simulink model "Task2"  (R2018a)
settings: Solver=FixedStepAuto  StartTime=0.0  StopTime=20  FixedStep=0.01  RelTol=1e-3
libraries: fl_lib x11, nesl_utility x7, simulink x3, elec_lib x3, sdl_lib x1
settings Model: Creator=Archana  LastModifiedBy=samak

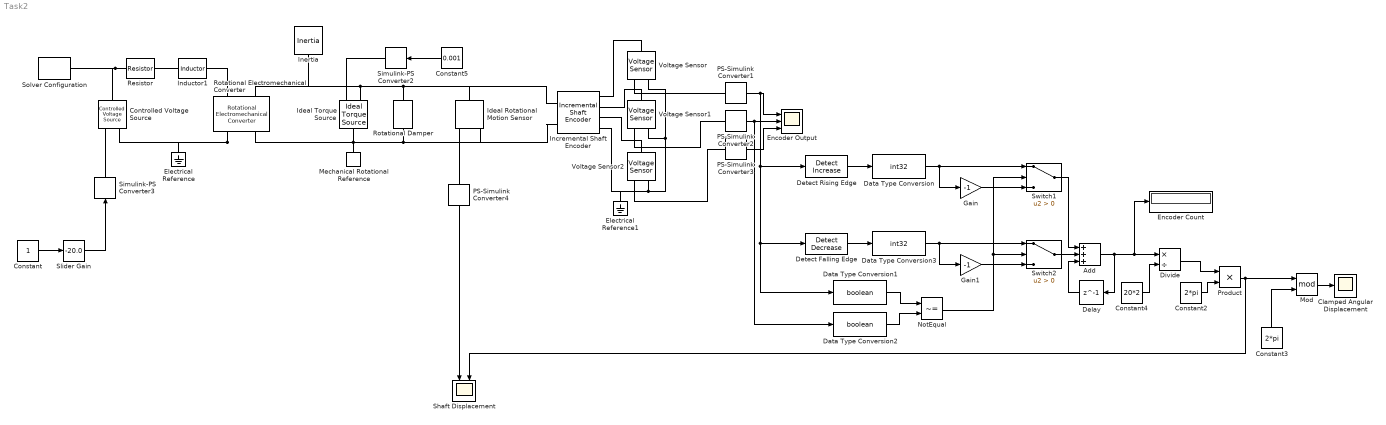
== system Task2 ==
  Add : Sum  Inputs=+++
  Clamped Angular Displacement : Scope
  "Constant " : Constant
  Constant2 : Constant  Value=2*pi
  Constant3 : Constant  Value=2*pi
  Constant4 : Constant  Value=20*2
  Constant5 : Constant  Value=0.001
  "Controlled Voltage Source " : fl_lib/Electrical/Electrical Sources/Controlled Voltage Source
  Data Type Conversion : DataTypeConversion  OutDataTypeStr=int32
  Data Type Conversion1 : DataTypeConversion  OutDataTypeStr=boolean
  Data Type Conversion2 : DataTypeConversion  OutDataTypeStr=boolean
  Data Type Conversion3 : DataTypeConversion  OutDataTypeStr=int32
  Delay : Delay  DelayLength=1
  Detect Falling Edge : simulink/Logic and Bit Operations/Detect Decrease  vinit=0.0  OutDataTypeStr=boolean
  Detect Rising Edge : simulink/Logic and Bit Operations/Detect Increase  vinit=0.0  OutDataTypeStr=boolean
  Divide : Product  Inputs=*/
  "Electrical Reference " : fl_lib/Electrical/Electrical Elements/Electrical Reference
  Electrical Reference1 : fl_lib/Electrical/Electrical Elements/Electrical Reference
  Encoder Count : Display
  Encoder Output : Scope  NumInputPorts=3
  Gain : Gain  Gain=-1
  Gain1 : Gain  Gain=-1
  "Ideal Torque Source " : fl_lib/Mechanical/Mechanical Sources/Ideal Torque Source
  "Ideal Rotational Motion Sensor " : fl_lib/Mechanical/Mechanical Sensors/Ideal Rotational Motion Sensor  offset=0 rad
  Incremental Shaft Encoder : elec_lib/Sensors/Incremental Shaft Encoder  NPulse=20  Vm=1 V  angle0=0 deg
      settings: SourceProductName=Simscape Electronics  SourceProductBaseCode=SN
  Inductor1 : elec_lib/Passive Devices/Inductor  l=0.5 H  L_tol=20  enable_L_tol=0  tol_distribution=1  nSigma=4  r=0 Ohm  g=1e-9 1/Ohm  enable_operating_limits=0  operating_limit_action=2  max_working_current=1 A  power_rating=1 W  enable_faults=0  fault_action=1  lambdaPercent=50  k_faulted=0.9999  turnsShort=0  openCct=0  groundShort=0  groundShortG=0 1/Ohm  tau_fault=1e-3 s  enable_temporal_fault=0  t_fault=1 s  enable_behavioral_fault=0  max_permissible_voltage=100 V  n_fail_on_voltage=1  max_permissible_current=1 A  t_fail_on_current=1 s  i_L_specify=off  i_L_priority=High  i_L=0 A  i_L_nominal_specify=off  i_L_nominal_unit=A  i_L_nominal_value=1
      settings: SourceProductName=Simscape Electronics  SourceProductBaseCode=SN
  "Inertia " : fl_lib/Mechanical/Rotational Elements/Inertia  inertia=0.01 kg*m^2  w_specify=off  w_priority=High  w=0 rad/s  w_nominal_specify=off  w_nominal_unit=rad/s  w_nominal_value=1  t_specify=off  t_priority=None  t=0 N*m  t_nominal_specify=off  t_nominal_unit=N*m  t_nominal_value=1
  "Mechanical Rotational Reference " : fl_lib/Mechanical/Rotational Elements/Mechanical Rotational Reference
  Mod : Math  Operator=mod  SaturateOnIntegerOverflow=on
  NotEqual : RelationalOperator  Operator=~=  OutDataTypeStr=boolean  RndMeth=Simplest
  PS-Simulink Converter{1..4} (4 alike) : nesl_utility/PS-Simulink Converter  PhysicalDomain=network_engine_domain  SubClassName=ps_output  LeftPortType=input  RightPortType=output  PseudoPeriodic=off  Frequencies=[]  Unit=1  AffineConversion=off
  Product : Product
  "Resistor " : elec_lib/Passive Devices/Resistor  R=1 Ohm  R_tol=5  enable_R_tol=0  tol_distribution=1  nSigma=4  enable_operating_limits=0  operating_limit_action=2  max_working_voltage=100 V  power_rating=1 W  enable_faults=0  fault_action=1  R_faulted=inf Ohm  enable_temporal_fault=0  t_fault=1 s  enable_behavioral_fault=0  max_permissible_current=1 A  t_fail_on_current=1 s  noise_mode=0  sample_time=1e-3 s  repeatability=1  auto_seed=4168664255  user_seed=0  Tdevice=25 degC  alpha=3.93e-3 1/K  Tmeas=25 degC  thermal_mass=100 J/K  power_derating_T1=70 degC  power_derating_T2=155 degC  operating_temperature_range_vec=[-50, 150] degC  temperature_specify=off  temperature_priority=High  temperature=298.15 K  temperature_nominal_specify=off  temperature_nominal_unit=K  temperature_nominal_value=1
  "Rotational Damper " : sdl_lib/Couplings & Drives/Springs & Dampers/Rotational Damper  D=0.1 N*m/(rad/s)  enable_faults=0  b_fault=100 N*m/(rad/s)  temporal_fault=0  fault_time=5 s  shock_fault=0  acceleration_limit=100 rad/s^2  shock_limit=1  report_fault=1
      settings: SourceProductName=Simscape Driveline  SourceProductBaseCode=LD
  "Rotational Electromechanical Converter " : fl_lib/Electrical/Electrical Elements/Rotational Electromechanical Converter  K=0.01 V/(rad/s)  i_specify=off  i_priority=None  i=0 A  i_nominal_specify=off  i_nominal_unit=A  i_nominal_value=1  v_specify=off  v_priority=None  v=0 V  v_nominal_specify=off  v_nominal_unit=V  v_nominal_value=1  t_specify=off  t_priority=None  t=0 N*m  t_nominal_specify=off  t_nominal_unit=N*m  t_nominal_value=1  w_specify=off  w_priority=None  w=0 rad/s  w_nominal_specify=off  w_nominal_unit=rad/s  w_nominal_value=1
      settings: SourceProductName=Simscape
  Shaft Displacement : Scope  NumInputPorts=2
  Simulink-PS Converter2 : nesl_utility/Simulink-PS Converter  PhysicalDomain=network_engine_domain  SubClassName=ps_input  LeftPortType=input  RightPortType=output  PseudoPeriodic=off  Frequencies=[]  NoiseDistribution=none  NoiseParameters=[]  Unit=1  AffineConversion=off  FilteringAndDerivatives=provide  SimscapeFilterOrder=1  InputFilterTimeConstant=0.001  UdotUserProvided=0
  Simulink-PS Converter3 : nesl_utility/Simulink-PS Converter  PhysicalDomain=network_engine_domain  SubClassName=ps_input  LeftPortType=input  RightPortType=output  PseudoPeriodic=off  Frequencies=[]  NoiseDistribution=none  NoiseParameters=[]  Unit=1  AffineConversion=off  FilteringAndDerivatives=provide  SimscapeFilterOrder=1  InputFilterTimeConstant=0.001  UdotUserProvided=0
  "Slider Gain " : simulink/Math Operations/Slider Gain  gain=-20.0  low=-20  high=20
  "Solver Configuration " : nesl_utility/Solver Configuration  PhysicalDomain=network_engine_domain  SubClassName=solver  LeftPortType=input  RightPortType=generic  Tones=[]  Harmonics=[]  SimulateNoise=off  Profile=off  UseLocalSampling=off  EnableSwitchedLinearOptims=on  FrequencyDomain=off  UseCCode=off  RelTol=0.001  AbsTol=1e-06  MinStep=1e-09  ToWorkspace=off  RevertToSquareIcSolve=off  NumHomotopyIterations=100  PhasorMode=off  PhasorModeNumHarmonics=1  DoDC=off  ResidualTolerance=1e-09  UseLocalSolver=off  LocalSolverChoice=NE_BACKWARD_EULER_ADVANCER  LocalSolverSampleTime=0.001  DoFixedCost=off  MaxNonlinIter=3  MaxModeIter=2  LinearAlgebra=Sparse  EquationFormulation=NE_TIME_EF  DelaysMemoryBudget=1024  AutomaticFiltering=on  FilteringTimeConstant=0.001
  "Switch1 " : Switch  Criteria=u2 > Threshold
  "Switch2 " : Switch  Criteria=u2 > Threshold
  Voltage Sensor : fl_lib/Electrical/Electrical Sensors/Voltage Sensor
  Voltage Sensor1 : fl_lib/Electrical/Electrical Sensors/Voltage Sensor
  Voltage Sensor2 : fl_lib/Electrical/Electrical Sensors/Voltage Sensor
  wires:
  PS-Simulink Converter1/1 -> Encoder Output/1, Detect Rising Edge/1, Detect Falling Edge/1, Data Type Conversion1/1
  PS-Simulink Converter2/1 -> Data Type Conversion2/1, Encoder Output/2
  PS-Simulink Converter3/1 -> Encoder Output/3
  Data Type Conversion/1 -> Gain/1, "Switch1 "/1
  Gain/1 -> "Switch1 "/3
  "Switch1 "/1 -> Add/1
  Delay/1 -> Add/3
  Add/1 -> Encoder Count/1, Divide/1, Delay/1
  Constant4/1 -> Divide/2
  Divide/1 -> Product/1
  Constant2/1 -> Product/2
  Detect Rising Edge/1 -> Data Type Conversion/1
  Data Type Conversion2/1 -> NotEqual/2
  NotEqual/1 -> "Switch2 "/2, "Switch1 "/2
  Product/1 -> Mod/1, Shaft Displacement/2
  Constant3/1 -> Mod/2
  Mod/1 -> Clamped Angular Displacement/1
  Data Type Conversion1/1 -> NotEqual/1
  Detect Falling Edge/1 -> Data Type Conversion3/1
  "Switch2 "/1 -> Add/2
  Data Type Conversion3/1 -> Gain1/1, "Switch2 "/1
  Gain1/1 -> "Switch2 "/3
  "Constant "/1 -> "Slider Gain "/1
  "Slider Gain "/1 -> Simulink-PS Converter3/1
  Constant5/1 -> Simulink-PS Converter2/1
  PS-Simulink Converter4/1 -> Shaft Displacement/1
  connections:
  Voltage Sensor2/RConn2 -- Incremental Shaft Encoder/RConn4 -- Electrical Reference1/LConn1 -- Voltage Sensor1/RConn2 -- Voltage Sensor/RConn2
  Voltage Sensor/LConn1 -- Incremental Shaft Encoder/RConn1
  Voltage Sensor1/LConn1 -- Incremental Shaft Encoder/RConn2
  Voltage Sensor2/LConn1 -- Incremental Shaft Encoder/RConn3
  Voltage Sensor/RConn1 -- PS-Simulink Converter1/LConn1
  Voltage Sensor1/RConn1 -- PS-Simulink Converter2/LConn1
  Voltage Sensor2/RConn1 -- PS-Simulink Converter3/LConn1
  "Rotational Damper "/LConn1 -- Incremental Shaft Encoder/LConn1 -- "Ideal Rotational Motion Sensor "/LConn1 -- "Ideal Torque Source "/RConn2 -- "Rotational Electromechanical Converter "/LConn2 -- "Inertia "/LConn1
  "Rotational Electromechanical Converter "/RConn1 -- "Controlled Voltage Source "/RConn2 -- "Electrical Reference "/LConn1
  "Ideal Torque Source "/LConn1 -- "Rotational Damper "/RConn1 -- Incremental Shaft Encoder/LConn2 -- "Ideal Rotational Motion Sensor "/RConn1 -- "Rotational Electromechanical Converter "/RConn2 -- "Mechanical Rotational Reference "/LConn1
  "Resistor "/LConn1 -- "Controlled Voltage Source "/LConn1 -- "Solver Configuration "/RConn1
  Inductor1/LConn1 -- "Resistor "/RConn1
  PS-Simulink Converter4/LConn1 -- "Ideal Rotational Motion Sensor "/RConn3
  Simulink-PS Converter2/RConn1 -- "Ideal Torque Source "/RConn1
  "Rotational Electromechanical Converter "/LConn1 -- Inductor1/RConn1
  Simulink-PS Converter3/RConn1 -- "Controlled Voltage Source "/RConn1
